simulink model "DC_modelling_control"  (R2022b)
settings: Solver=VariableStepAuto  StartTime=0.0  StopTime=100  FixedStep=1e-6  MaxStep=1e-4  RelTol=1e-3
values from neighbouring files (symbols this model uses):
  B_nom = 0.05    [PID_tuning.m]
  J_nom = 2.0    (= 2)    [PID_tuning.m]
  Kb_nom = 1.0    (= 1)    [PID_tuning.m]
  Kt_nom = 1.0    (= 1)    [PID_tuning.m]
  L_nom = 0.5    [PID_tuning.m]
  R_nom = 0.2    [PID_tuning.m]
libraries: slpidlib x1
settings Model: Creator=nyinyia  LastModifiedBy=nyinyia

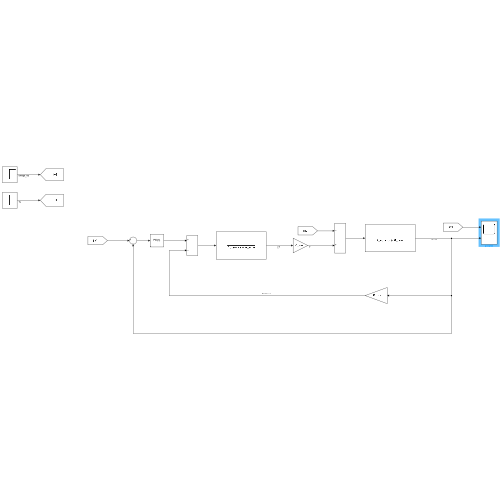
[thumbnail: Simulink's stored preview of the top-level diagram]
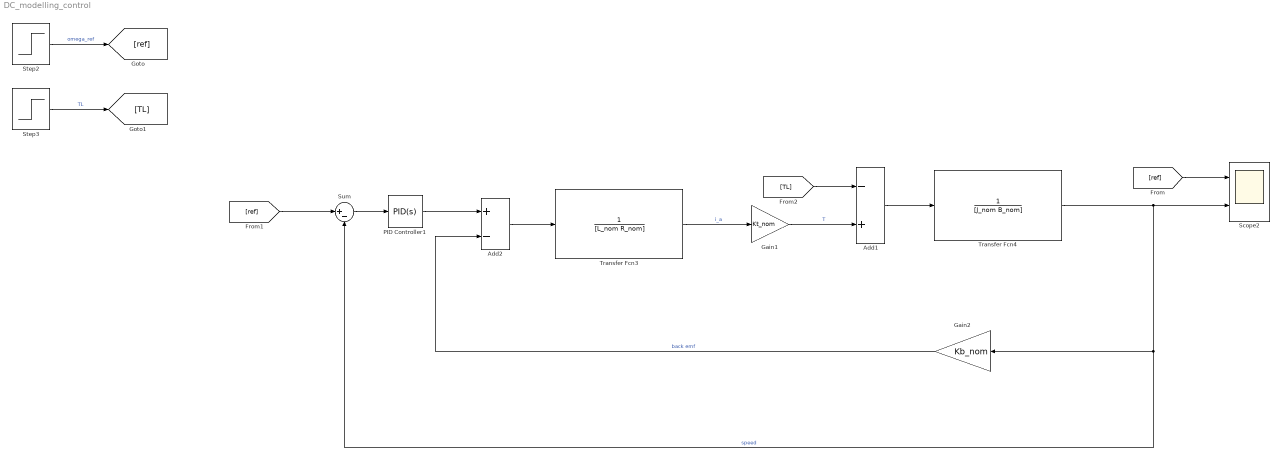
== system DC_modelling_control ==
  Add1 : Sum  Inputs=-+
  Add2 : Sum  Inputs=+-
  Gain1 : Gain  Gain=Kt_nom
  Gain2 : Gain  Gain=Kb_nom
  PID Controller1 : slpidlib/PID Controller  Controller=PID  Form=Parallel  TimeDomain=Continuous-time  UseExternalTs=off  SampleTime=-1  IntegratorMethod=Forward Euler  FilterMethod=Forward Euler  ControllerParametersSource=internal  P=3.33648935332675  I=0.656107950597057  UseKiTs=off  D=-0.0141651780403183  N=235.541646128988  UseFilter=on  TunerSelectOption=Transfer Function Based (PID Tuner App)  InitialConditionSource=internal  InitialConditionForIntegrator=0  InitialConditionForFilter=0  DifferentiatorICPrevScaledInput=0  ExternalReset=none  TrackingMode=off  Kt=1  LimitOutput=off  SatLimitsSource=internal  UpperSaturationLimit=inf  LowerSaturationLimit=-inf  LinearizeAsGain=on  AntiWindupMode=none  Kb=1  LimitIntegrator=off  UpperIntegratorSaturationLimit=inf  LowerIntegratorSaturationLimit=-inf  POutMin=[]  POutMax=[]  IOutMin=[]  IOutMax=[]  DOutMin=[]  DOutMax=[]  NOutMin=[]  NOutMax=[]  SumOutMin=[]  SumOutMax=[]  SaturationOutMin=[]  SaturationOutMax=[]  PParamMin=[]  PParamMax=[]  IParamMin=[]  IParamMax=[]  DParamMin=[]  DParamMax=[]  NParamMin=[]  NParamMax=[]  KbParamMin=[]  KbParamMax=[]  KtParamMin=[]  KtParamMax=[]  KbOutMin=[]  KbOutMax=[]  KtOutMin=[]  KtOutMax=[]  IntegratorOutMin=[]  IntegratorOutMax=[]  FilterOutMin=[]  FilterOutMax=[]  SumI1OutMin=[]  SumI1OutMax=[]  SumI2OutMin=[]  SumI2OutMax=[]  SumI3OutMin=[]  SumI3OutMax=[]  SumI4OutMin=[]  SumI4OutMax=[]  SumDOutMin=[]  SumDOutMax=[]  DifferentiatorOutMin=[]  DifferentiatorOutMax=[]  FilterDiffOutCoefMin=[]  FilterDiffOutCoefMax=[]  ReciprocalOutMin=[]  ReciprocalOutMax=[]  SumDenOutMin=[]  SumDenOutMax=[]  SumNumOutMin=[]  SumNumOutMax=[]  DivideOutMin=[]  DivideOutMax=[]  UdiffTsProdOutMin=[]  UdiffTsProdOutMax=[]  NTsProdOutMin=[]  NTsProdOutMax=[]  UintegralTsProdOutMin=[]  UintegralTsProdOutMax=[]  UngainTsProdOutMin=[]  UngainTsProdOutMax=[]  ClampingZeroOutDataTypeStr=Inherit: Inherit via back propagation  ClampingZeroOutMin=[]  ClampingZeroOutMax=[]  FilterDenConstantOutDataTypeStr=Inherit: Inherit via back propagation  FilterDenConstantOutMin=[]  FilterDenConstantOutMax=[]  PCopyOutDataTypeStr=Inherit: Inherit via back propagation  PCopyOutMin=[]  PCopyOutMax=[]  NCopyOutDataTypeStr=Inherit: Inherit via back propagation  NCopyOutMin=[]  NCopyOutMax=[]  IntegratorContinuousStateAttributes=''  IntegratorStateMustResolveToSignalObject=off  IntegratorRTWStateStorageClass=Auto  FilterContinuousStateAttributes=''  FilterStateMustResolveToSignalObject=off  FilterRTWStateStorageClass=Auto  ParallelPVariant=InternalParameters  IdealPVariant=Disabled  IVariant=InternalParameters  DVariant=InternalParameters  IntegratorVariant=Continuous  SatVariant=Disabled  AWVariant=Passthrough  PCopyVariant=Disabled  TRVariant=Disabled  FdbkBlocksVariant=Forward  IdealPFdbkVariant=Disabled  SatFdbkVariant=Disabled  DerivativeFilterVariant=ContFilter  NVariant=InternalParameters  NCopyVariant=Disabled  FilterICVariant=InternalICsFilter  IntegratorICVariant=InternalICs  ExternalResetVariant=Disabled  TRSumVariant=Passthrough  SumFdbkVariant=Disabled  SumVariant=Sum_PID  TsampFilterVariant=InternalTs  TsampNgainVariant=Passthrough  TsampIntegralVariant=Passthrough  ExternalSaturationOutDataTypeStr=Inherit: Same as second input
  Scope2 : Scope  NumInputPorts=2
  Step2 : Step  Time=0.1  After=80  SampleTime=0
  Step3 : Step  Time=75  After=20  SampleTime=0
  Sum : Sum  Inputs=|+-
  Transfer Fcn3 : TransferFcn  Denominator=[L_nom R_nom]
  Transfer Fcn4 : TransferFcn  Denominator=[J_nom B_nom]
  wires:
  Transfer Fcn4/1 -> Gain2/1, Sum/2, Scope2/2  "speed"
  Transfer Fcn3/1 -> Gain1/1  "i_a"
  Add2/1 -> Transfer Fcn3/1
  Gain2/1 -> Add2/2  "back emf"
  Gain1/1 -> Add1/2  "T"
  Step2/1 -> [ref]  "omega_ref"
  Sum/1 -> PID Controller1/1
  PID Controller1/1 -> Add2/1
  Add1/1 -> Transfer Fcn4/1
  [ref] -> Scope2/1
  [ref] -> Sum/1
  Step3/1 -> [TL]  "TL"
  [TL] -> Add1/1
